simulink model "flightControlSystem2"  (R2019a)
settings: Solver=ode3  StartTime=0  StopTime=TFinal  FixedStep=Ts  RelTol=1e-3  EnableMultiTasking=on
InitFcn:
  | %生成模板
  | temp_Image = uint8(ones(120,160));
  | 
  | [m,n] = size(temp_Image);
  | angle = 10*pi/180;
  | 
  | left_point = 70;
  | right_point = 90;
  | j = 71;
  | for i = 1:50
  |     temp_left_point = floor(left_point - i*sin(angle));
  |     temp_right_point = floor(right_point + i*sin(angle));
  |     if temp_left_point < 1
  |         temp_left_point = 1;
  |     end
  |     if temp_right_point > 180
  |         temp_right_point = 180;
  |     end
  |     temp_Image(j,temp_left_point:temp_right_point) = 0;
  |     j = j+1;
  | end
undefined symbols (not defined in the file): codertarget, Controller, DiscIntNeverNeededParam, Discrete, Estimator, g, gray, init, pos_ref, Sensors, takeoff_flag, Time, Ts, Vehicle
libraries: simulink x60, visiontransforms x4, sharedtransform x3, ctrlSharedLib x2, visionsinks x2, sharedutil x1, visionanalysis x1, parrotlib x1
(part 3 of 3)

== matlab function flightControlSystem2/Control System/Path Planning/state_control ==
  data: line_sum_angle input; line_target input; line_flag input; drone_targetout output; circle_output input; drone_angle output; circle_flag input; drone_xyz input; yaw input; F1 data_store_memory; F2 data_store_memory; F3 data_store_memory
function [drone_targetout, drone_angle] = state_control(line_sum_angle, line_target, line_flag, circle_output, circle_flag, drone_xyz, yaw)

global F1 F2 F3

if line_flag == -1 && circle_flag ~= -1 && F1 ~= 2
    F1 = 1;
end

    
if F1 == 0
    % follow the line
    drone_target = line_target;
    drone_angle = line_sum_angle;
    target = [0,0,0]';
    sum_x = 0;
    sum_y = 0;
elseif F1 == 1
    % move toward the center of circle
    circle_output(1,1) = 160 - circle_output(1,1);
    circle_output(1,2) = 120 - circle_output(1,2);
    sum_y = circle_output(1,1)-80;
    sum_x = 60-circle_output(1,2);
     sum_x = sum_x;
     sum_y = -sum_y;
    temp = sqrt(sum_x^2 + sum_y^2);
    sum_x = sum_x/temp;
    sum_y = sum_y/temp;
    
    target = 0.15*9.4e-3*[sum_x;sum_y;0];
	distance = temp;
    
    drone_target = drone_xyz + target;
    drone_angle = double(yaw);
    
    if distance < 15
    F2  = F2 + 1;
    if F2 >= 1
       F1 = 2;
       F3 = drone_target;
    end
    
    end
    down = 0;
    drone_target(3) = drone_target(3) + down;
    
elseif F1 ==2
    % move down
    if circle_flag ~= -1
    circle_output(1,1) = 160 - circle_output(1,1);
    circle_output(1,2) = 120 - circle_output(1,2);
    sum_y = circle_output(1,1)-80;
    sum_x = 60-circle_output(1,2);
         sum_x = sum_x;
         sum_y = -sum_y;
        temp = sqrt(sum_x^2 + sum_y^2);
        sum_x = sum_x/temp;
        sum_y = sum_y/temp;

        target = 0.1*9.4e-3*[sum_x;sum_y;0];

%         if drone_xyz(3)>-0.5
%             target = [0,0,0]';
%         end
        
        drone_target = drone_xyz + target;
        drone_target = (drone_target + F3)/2;
        F3 = drone_target;
    else
        drone_target = F3;
    end
    
    sum_x = 0;
    sum_y = 0;
    
    drone_angle = double(yaw);
    drone_target = F3;

    down = 0.1;
    drone_target(3) = drone_target(3) + down;
    
% 	if drone_xyz(3)>-0.5
%         target = 0;
%     end
    
     F3 = drone_target;

else
    sum_x = 0;
    sum_y = 0;
    target = [0,0,0]';
    drone_target = F3;
    drone_angle = double(yaw);
end

drone_targetout = drone_target;
xxx = F2;
yyy = circle_flag;
ob1 = [sum_x,sum_y];

== matlab function flightControlSystem2/Control System/Path Planning/three_circles_control ==
  data: image_control_data input; drone_xyz input; line_sum_angle output; A1 data_store_memory; A3 data_store_memory; A2 data_store_memory; line_target output; yaw input; A4 data_store_memory; FLAG data_store_memory; index_model data_store_memory; B1 data_store_memory; B2 data_store_memory; B3 data_store_memory; B4 data_store_memory
function [line_sum_angle, line_target] = three_circles_control(image_control_data, drone_xyz, yaw)
Conv_coeff = image_control_data(1);
line_angle = image_control_data(2);

%% 定义
global A1 A2 A3 A4 FLAG index_model
global B1 B2 B3 B4

%% 角度
 line_angle = line_angle*0.7 + A1*0.1 + A2*0.1 + A3*0.1;
%%
% if abs(line_angle) > 1.5 
%     line_angle = 1.5;
% elseif abs(line_angle) <0.05
%     line_angle = 0;
% end

%% 分级调参
% 


% 一级档
if abs(line_angle) < 0.1
    angle_change = 0.15;
    speed_change = 7;
    
% 二级档
elseif abs(line_angle) < 0.2
   angle_change = 0.40;
   speed_change = 5.5;
   
% 三级档
elseif abs(line_angle) < 0.6
    angle_change = 0.5;
    speed_change = 3;
    
% 四级档
elseif abs(line_angle) < 1.2
    angle_change = 0.5;
    speed_change = 3;
    
% 五级档  
else 
    angle_change = 0.55;
    speed_change = 3;
    
end 

% speed_change = speed_change*0.8 + B1*0.1 + B2*0.1 ;

%% 1 + B3*0.1 + B4*0.1
% if abs(line_angle) < 0.1
%     angle_change = 0.15;
%     speed_change = 7;
%     
% % 二级档
% elseif abs(line_angle) < 0.4
%    angle_change = 0.40;
%    speed_change = 6;
   

%% 3

% % 一级档
% if abs(line_angle) < 0.1
%     angle_change = 0.15;
%     speed_change = 7;
%     
% % 二级档
% elseif abs(line_angle) < 0.2
%    angle_change = 0.40;
%    speed_change = 6;
%    
% % 三级档
% elseif abs(line_angle) < 0.6
%     angle_change = 0.5;
%     speed_change = 3;
%     
% % 四级档
% elseif abs(line_angle) < 1.2
%     angle_change = 0.5;
%     speed_change = 3;
%     
% % 五级档  
% else 
%     angle_change = 0.55;
%     speed_change = 3;
%     
% end 


% % 一级档
% if abs(line_angle) < 0.1
%     angle_change = 0.2;
%     speed_change = 7;
%     
% % 二级档
% elseif abs(line_angle) < 0.2
%    angle_change = 0.3;
%    speed_change = 7;
%    
% % 三级档
% elseif abs(line_angle) < 0.5
%     angle_change = 0.45;
%     speed_change = 3;
%     
% % 四级档
% elseif abs(line_angle) < 0.7
%     angle_change = 0.65;
%     speed_change = 4;
%     
% % 五级档  
% else 
%     angle_change = 0.55;
%     speed_change = 5;
%     
% end 

%%

% %% 分级调参
% % 
% 
% 
% % 一级档
% if abs(line_angle) < 0.1
%     angle_change = 0.15;
%     speed_change = 9;
%     
% % 二级档
% elseif abs(line_angle) < 0.2
%    angle_change = 0.25;
%    speed_change = 7;
%    
% % 三级档
% elseif abs(line_angle) < 0.6
%     angle_change = 0.35;
%     speed_change = 6;
%     
% % 四级档
% elseif abs(line_angle) < 0.7
%     angle_change = 0.45;
%     speed_change = 5;
%     
% % 五级档  
% else 
%     angle_change = 0.55;
%     speed_change = 5;
%     
% end 
%%
%% 函数调参
% angle_change = 0.667*abs(angle);
% speed_change = k*angle_change+ b;



%% 控制
if abs(drone_xyz(3)+1.1) > 0.1
    angle_change = 1;
end

sum_angle = double(yaw)+ angle_change *line_angle;

sum_x = cos(sum_angle);
sum_y = sin(sum_angle);
target = speed_change*Conv_coeff*[sum_x;sum_y;0];
target = drone_xyz + target;

% target(3) = -1.1;
if target(3) >= -1.1
    target(3) = target(3) - 0.1;
end

if abs(drone_xyz(3)+1.1) > 0.1
    target(1) = 0;
    target(2) = 0;
    
end
%     

%% 更新
A3 = A2;
A2 = A1;
A1 = line_angle;

B4 = B3;
B3 = B2;
B2 = B1;
B1 = speed_change;

line_sum_angle = sum_angle;
line_target = target;

== matlab function flightControlSystem2/Control System/Path Planning2/line_gravity_point ==
  data: Conv_coeff output; image_data input; A1 data_store_memory; A3 data_store_memory; A2 data_store_memory; center_gravity_area output; line_flag output
function [Conv_coeff,center_gravity_area,line_flag]  = center_gravity(image_data)
%% 找红色
r = image_data(1);
g = image_data(2);
b = image_data(3);
flag = 1;
Image = r;
index = g(:)>50 | b(:)>50;
Image(index) = 0;
Image = Image.*temp_Image;
[width,height] = size(Image);

%% 找路径
skeletonizedImage = bwmorph(Image, 'thin', inf);
edgeImage = bwperim(Image);
Image2 = bwperim(skeletonizedImage);

%% 求出转换系数
%等分处理,取众数，求出路宽,
%需要从图像的x,y方向上进行截取的原因是，为了保证无人机能转弯。
%因为后面求出了转换系数，只考虑x方向的话，到转弯处，转换系数会发现剧烈变化，从而影响输出。
% temp = zeros(26,1);
% k = 1;
% for i = 10:10:width-10 %水平方向取11个值
%     index = find(edgeImage(i,:) == 1);
%     if ~isempty(index)
%         temp(k) = max(index) - min(index);
%     else
%         temp(k) = k;
%     end
%      k = k+1;
% end
% for i = 10:10:height-10 %垂直方向取15个值
%     index = find(edgeImage(:,i) == 1);
%     if ~isempty(index)
%         temp(k) = max(index) - min(index);
%     else
%         temp(k) = k;
%     end
%      k = k+1;
% end
% road_image_length = mode(temp);
% 
% %转换系数，即真实距离与图像像素距离之比,一个像素对应的实际距离
% Conv_coeff = 0.15/road_image_length;
% if Conv_coeff > 0.01
%     Conv_coeff = 0.01;
% end
Conv_coeff = 9.4e-3;
%% 跟踪算法
Image_roi = Image2;
center_x = 60;
center_y = 80;

%%


cut = [45;50;55];

cut_XY = zeros(length(cut(:)),4);
for i = 1:length(cut_XY(:,1))
    cut_XY(i,1) = center_x - cut(i);
    cut_XY(i,2) = center_y - cut(i);
    cut_XY(i,3) = center_x + cut(i);
    cut_XY(i,4) = center_y + cut(i);
end

sum_vector = zeros(length(cut(:)),3);

for i = 1:length(cut_XY(:,1))
    I1 = Image_roi(cut_XY(i,1):cut_XY(i,3),cut_XY(i,2):cut_XY(i,4));
    index = find(I1(:)==1);
    position = zeros(length(index),3);
    I1_center_x = 1+cut(i);
    I1_center_y = 1+cut(i);
    if ~isempty(index)
        for k=1:length(index)
            [position(k,1),position(k,2)] = ind2sub(size(I1),index(k));
            position(k,1) = I1_center_x - position(k,1);
            position(k,2) = position(k,2) - I1_center_y;
            position(k,3) = sqrt((position(k,1))^2+(position(k,2))^2);
        end
        index1 = position(:,3) <= cut(i)+0.5 & position(:,3) >= cut(i)-0.5 & position(:,1) > 0;
        position = position(index1,:);
    end
    if ~isempty(index)
        if length(position(:,1))==1
            sum_vector(i,1) = position(1,1);
            sum_vector(i,2) = position(1,2);
            temp = sqrt(sum_vector(i,1)^2 + sum_vector(i,2)^2);
            sum_vector(i,1) = sum_vector(i,1)/temp;
            sum_vector(i,2) = sum_vector(i,2)/temp;
            sum_vector(i,3) = atan2(sum_vector(i,2),sum_vector(i,1));
        end
    end
end
% vector = 0.25*sum_vector(1,:)+0.5*sum_vector(2,:)+0.25*sum_vector(3,:);
vector = 0.3*sum_vector(1,:)+0.3*sum_vector(2,:)+0.4*sum_vector(3,:);
if abs(sum_vector(1,1)) < 1e-5 && abs(sum_vector(1,2)) < 1e-5
    flag = -1;
end
line = vector(3);
line_flag = flag;

== matlab function flightControlSystem2/Control System/Path Planning1/state_control ==
  data: center_gravity_point input; line_target input; line_flag input; drone_targetout output; circle_output input; drone_angle output; circle_flag input; drone_xyz input; yaw input; F1 data_store_memory; F2 data_store_memory; F3 data_store_memory
function [drone_targetout, drone_angle] = state_control(center_gravity_point, line_target, line_flag, circle_output, circle_flag, drone_xyz, yaw)

global F1 F2 F3

if line_flag == -1 && circle_flag ~= -1 && F1 ~= 2
    F1 = 1;
end

    
if F1 == 0
    % follow the line
    drone_target = line_target;
    drone_angle = line_sum_angle;
    target = [0,0,0]';
    sum_x = 0;
    sum_y = 0;
elseif F1 == 1
    % move toward the center of circle
    circle_output(1,1) = 160 - circle_output(1,1);
    circle_output(1,2) = 120 - circle_output(1,2);
    sum_y = circle_output(1,1)-80;
    sum_x = 60-circle_output(1,2);
     sum_x = sum_x;
     sum_y = -sum_y;
    temp = sqrt(sum_x^2 + sum_y^2);
    sum_x = sum_x/temp;
    sum_y = sum_y/temp;
    
    target = 0.15*9.4e-3*[sum_x;sum_y;0];
	distance = temp;
    
    drone_target = drone_xyz + target;
    drone_angle = double(yaw);
    
    if distance < 15
    F2  = F2 + 1;
    if F2 >= 1
       F1 = 2;
       F3 = drone_target;
    end
    
    end
    down = 0;
    drone_target(3) = drone_target(3) + down;
    
elseif F1 ==2
    % move down
    if circle_flag ~= -1
    circle_output(1,1) = 160 - circle_output(1,1);
    circle_output(1,2) = 120 - circle_output(1,2);
    sum_y = circle_output(1,1)-80;
    sum_x = 60-circle_output(1,2);
         sum_x = sum_x;
         sum_y = -sum_y;
        temp = sqrt(sum_x^2 + sum_y^2);
        sum_x = sum_x/temp;
        sum_y = sum_y/temp;

        target = 0.1*9.4e-3*[sum_x;sum_y;0];

%         if drone_xyz(3)>-0.5
%             target = [0,0,0]';
%         end
        
        drone_target = drone_xyz + target;
        drone_target = (drone_target + F3)/2;
        F3 = drone_target;
    else
        drone_target = F3;
    end
    
    sum_x = 0;
    sum_y = 0;
    
    drone_angle = double(yaw);
    drone_target = F3;

    down = 0.1;
    drone_target(3) = drone_target(3) + down;
    
% 	if drone_xyz(3)>-0.5
%         target = 0;
%     end
    
     F3 = drone_target;

else
    sum_x = 0;
    sum_y = 0;
    target = [0,0,0]';
    drone_target = F3;
    drone_angle = double(yaw);
end

drone_targetout = drone_target;
xxx = F2;
yyy = circle_flag;
ob1 = [sum_x,sum_y];

== matlab function flightControlSystem2/Control System/Path Planning1/center_gravity_control ==
  data: image_control_data input; drone_xyz input; center_gravity_point output; A1 data_store_memory; A3 data_store_memory; A2 data_store_memory; line_target output; yaw input; A4 data_store_memory; FLAG data_store_memory; index_model data_store_memory; B1 data_store_memory; B2 data_store_memory; B3 data_store_memory; B4 data_store_memory
function [center_gravity_point, line_target] = center_gravity_control(image_control_data, drone_xyz, yaw)
Conv_coeff = image_control_data(1);
line_angle = image_control_data(2);

%% 定义
global A1 A2 A3 A4 FLAG index_model
global B1 B2 B3 B4

%% 角度
 line_angle = line_angle*0.7 + A1*0.1 + A2*0.1 + A3*0.1;
%%
% if abs(line_angle) > 1.5 
%     line_angle = 1.5;
% elseif abs(line_angle) <0.05
%     line_angle = 0;
% end

%% 分级调参
% 


% 一级档
if abs(line_angle) < 0.1
    angle_change = 0.15;
    speed_change = 7;
    
% 二级档
elseif abs(line_angle) < 0.2
   angle_change = 0.40;
   speed_change = 5.5;
   
% 三级档
elseif abs(line_angle) < 0.6
    angle_change = 0.5;
    speed_change = 3;
    
% 四级档
elseif abs(line_angle) < 1.2
    angle_change = 0.5;
    speed_change = 3;
    
% 五级档  
else 
    angle_change = 0.55;
    speed_change = 3;
    
end 

% speed_change = speed_change*0.8 + B1*0.1 + B2*0.1 ;

%% 1 + B3*0.1 + B4*0.1
% if abs(line_angle) < 0.1
%     angle_change = 0.15;
%     speed_change = 7;
%     
% % 二级档
% elseif abs(line_angle) < 0.4
%    angle_change = 0.40;
%    speed_change = 6;
   

%% 3

% % 一级档
% if abs(line_angle) < 0.1
%     angle_change = 0.15;
%     speed_change = 7;
%     
% % 二级档
% elseif abs(line_angle) < 0.2
%    angle_change = 0.40;
%    speed_change = 6;
%    
% % 三级档
% elseif abs(line_angle) < 0.6
%     angle_change = 0.5;
%     speed_change = 3;
%     
% % 四级档
% elseif abs(line_angle) < 1.2
%     angle_change = 0.5;
%     speed_change = 3;
%     
% % 五级档  
% else 
%     angle_change = 0.55;
%     speed_change = 3;
%     
% end 


% % 一级档
% if abs(line_angle) < 0.1
%     angle_change = 0.2;
%     speed_change = 7;
%     
% % 二级档
% elseif abs(line_angle) < 0.2
%    angle_change = 0.3;
%    speed_change = 7;
%    
% % 三级档
% elseif abs(line_angle) < 0.5
%     angle_change = 0.45;
%     speed_change = 3;
%     
% % 四级档
% elseif abs(line_angle) < 0.7
%     angle_change = 0.65;
%     speed_change = 4;
%     
% % 五级档  
% else 
%     angle_change = 0.55;
%     speed_change = 5;
%     
% end 

%%

% %% 分级调参
% % 
% 
% 
% % 一级档
% if abs(line_angle) < 0.1
%     angle_change = 0.15;
%     speed_change = 9;
%     
% % 二级档
% elseif abs(line_angle) < 0.2
%    angle_change = 0.25;
%    speed_change = 7;
%    
% % 三级档
% elseif abs(line_angle) < 0.6
%     angle_change = 0.35;
%     speed_change = 6;
%     
% % 四级档
% elseif abs(line_angle) < 0.7
%     angle_change = 0.45;
%     speed_change = 5;
%     
% % 五级档  
% else 
%     angle_change = 0.55;
%     speed_change = 5;
%     
% end 
%%
%% 函数调参
% angle_change = 0.667*abs(angle);
% speed_change = k*angle_change+ b;



%% 控制
if abs(drone_xyz(3)+1.1) > 0.1
    angle_change = 1;
end

sum_angle = double(yaw)+ angle_change *line_angle;

sum_x = cos(sum_angle);
sum_y = sin(sum_angle);
target = speed_change*Conv_coeff*[sum_x;sum_y;0];
target = drone_xyz + target;

% target(3) = -1.1;
if target(3) >= -1.1
    target(3) = target(3) - 0.1;
end

if abs(drone_xyz(3)+1.1) > 0.1
    target(1) = 0;
    target(2) = 0;
    
end
%     

%% 更新
A3 = A2;
A2 = A1;
A1 = line_angle;

B4 = B3;
B3 = B2;
B2 = B1;
B1 = speed_change;

line_sum_angle = sum_angle;
line_target = target;

== matlab function flightControlSystem2/Control System/Path Planning2/state_control ==
  data: line_sum_angle input; line_flag input; drone_targetout output; circle_output input; drone_angle output; circle_flag input; drone_xyz input; yaw input; F1 data_store_memory; F2 data_store_memory; F3 data_store_memory
function [drone_targetout, drone_angle] = state_control(line_sum_angle, line_flag, circle_output, circle_flag, drone_xyz, yaw)

global F1 F2 F3

if line_flag == -1 && circle_flag ~= -1 && F1 ~= 2
    F1 = 1;
end

    
if F1 == 0
    % follow the line
    drone_target = line_target;
    drone_angle = line_sum_angle;
    target = [0,0,0]';
    sum_x = 0;
    sum_y = 0;
elseif F1 == 1
    % move toward the center of circle
    circle_output(1,1) = 160 - circle_output(1,1);
    circle_output(1,2) = 120 - circle_output(1,2);
    sum_y = circle_output(1,1)-80;
    sum_x = 60-circle_output(1,2);
     sum_x = sum_x;
     sum_y = -sum_y;
    temp = sqrt(sum_x^2 + sum_y^2);
    sum_x = sum_x/temp;
    sum_y = sum_y/temp;
    
    target = 0.15*9.4e-3*[sum_x;sum_y;0];
	distance = temp;
    
    drone_target = drone_xyz + target;
    drone_angle = double(yaw);
    
    if distance < 15
    F2  = F2 + 1;
    if F2 >= 1
       F1 = 2;
       F3 = drone_target;
    end
    
    end
    down = 0;
    drone_target(3) = drone_target(3) + down;
    
elseif F1 ==2
    % move down
    if circle_flag ~= -1
    circle_output(1,1) = 160 - circle_output(1,1);
    circle_output(1,2) = 120 - circle_output(1,2);
    sum_y = circle_output(1,1)-80;
    sum_x = 60-circle_output(1,2);
         sum_x = sum_x;
         sum_y = -sum_y;
        temp = sqrt(sum_x^2 + sum_y^2);
        sum_x = sum_x/temp;
        sum_y = sum_y/temp;

        target = 0.1*9.4e-3*[sum_x;sum_y;0];

%         if drone_xyz(3)>-0.5
%             target = [0,0,0]';
%         end
        
        drone_target = drone_xyz + target;
        drone_target = (drone_target + F3)/2;
        F3 = drone_target;
    else
        drone_target = F3;
    end
    
    sum_x = 0;
    sum_y = 0;
    
    drone_angle = double(yaw);
    drone_target = F3;

    down = 0.1;
    drone_target(3) = drone_target(3) + down;
    
% 	if drone_xyz(3)>-0.5
%         target = 0;
%     end
    
     F3 = drone_target;

else
    sum_x = 0;
    sum_y = 0;
    target = [0,0,0]';
    drone_target = F3;
    drone_angle = double(yaw);
end

drone_targetout = drone_target;
xxx = F2;
yyy = circle_flag;
ob1 = [sum_x,sum_y];

== matlab function flightControlSystem2/Control System/Path Planning2/random_points_control ==
  data: image_control_data input; drone_xyz input; random_point output; A1 data_store_memory; A3 data_store_memory; A2 data_store_memory; yaw input; A4 data_store_memory; FLAG data_store_memory; index_model data_store_memory; B1 data_store_memory; B2 data_store_memory; B3 data_store_memory; B4 data_store_memory
function random_point =  random_point_control(image_control_data, drone_xyz, yaw)
Conv_coeff = image_control_data(1);
line_angle = image_control_data(2);

%% 定义
global A1 A2 A3 A4 FLAG index_model
global B1 B2 B3 B4

%% 角度
 line_angle = line_angle*0.7 + A1*0.1 + A2*0.1 + A3*0.1;
%%
% if abs(line_angle) > 1.5 
%     line_angle = 1.5;
% elseif abs(line_angle) <0.05
%     line_angle = 0;
% end

%% 分级调参
% 


% 一级档
if abs(line_angle) < 0.1
    angle_change = 0.15;
    speed_change = 7;
    
% 二级档
elseif abs(line_angle) < 0.2
   angle_change = 0.40;
   speed_change = 5.5;
   
% 三级档
elseif abs(line_angle) < 0.6
    angle_change = 0.5;
    speed_change = 3;
    
% 四级档
elseif abs(line_angle) < 1.2
    angle_change = 0.5;
    speed_change = 3;
    
% 五级档  
else 
    angle_change = 0.55;
    speed_change = 3;
    
end 

% speed_change = speed_change*0.8 + B1*0.1 + B2*0.1 ;

%% 1 + B3*0.1 + B4*0.1
% if abs(line_angle) < 0.1
%     angle_change = 0.15;
%     speed_change = 7;
%     
% % 二级档
% elseif abs(line_angle) < 0.4
%    angle_change = 0.40;
%    speed_change = 6;
   

%% 3

% % 一级档
% if abs(line_angle) < 0.1
%     angle_change = 0.15;
%     speed_change = 7;
%     
% % 二级档
% elseif abs(line_angle) < 0.2
%    angle_change = 0.40;
%    speed_change = 6;
%    
% % 三级档
% elseif abs(line_angle) < 0.6
%     angle_change = 0.5;
%     speed_change = 3;
%     
% % 四级档
% elseif abs(line_angle) < 1.2
%     angle_change = 0.5;
%     speed_change = 3;
%     
% % 五级档  
% else 
%     angle_change = 0.55;
%     speed_change = 3;
%     
% end 


% % 一级档
% if abs(line_angle) < 0.1
%     angle_change = 0.2;
%     speed_change = 7;
%     
% % 二级档
% elseif abs(line_angle) < 0.2
%    angle_change = 0.3;
%    speed_change = 7;
%    
% % 三级档
% elseif abs(line_angle) < 0.5
%     angle_change = 0.45;
%     speed_change = 3;
%     
% % 四级档
% elseif abs(line_angle) < 0.7
%     angle_change = 0.65;
%     speed_change = 4;
%     
% % 五级档  
% else 
%     angle_change = 0.55;
%     speed_change = 5;
%     
% end 

%%

% %% 分级调参
% % 
% 
% 
% % 一级档
% if abs(line_angle) < 0.1
%     angle_change = 0.15;
%     speed_change = 9;
%     
% % 二级档
% elseif abs(line_angle) < 0.2
%    angle_change = 0.25;
%    speed_change = 7;
%    
% % 三级档
% elseif abs(line_angle) < 0.6
%     angle_change = 0.35;
%     speed_change = 6;
%     
% % 四级档
% elseif abs(line_angle) < 0.7
%     angle_change = 0.45;
%     speed_change = 5;
%     
% % 五级档  
% else 
%     angle_change = 0.55;
%     speed_change = 5;
%     
% end 
%%
%% 函数调参
% angle_change = 0.667*abs(angle);
% speed_change = k*angle_change+ b;



%% 控制
if abs(drone_xyz(3)+1.1) > 0.1
    angle_change = 1;
end

sum_angle = double(yaw)+ angle_change *line_angle;

sum_x = cos(sum_angle);
sum_y = sin(sum_angle);
target = speed_change*Conv_coeff*[sum_x;sum_y;0];
target = drone_xyz + target;

% target(3) = -1.1;
if target(3) >= -1.1
    target(3) = target(3) - 0.1;
end

if abs(drone_xyz(3)+1.1) > 0.1
    target(1) = 0;
    target(2) = 0;
    
end
%     

%% 更新
A3 = A2;
A2 = A1;
A1 = line_angle;

B4 = B3;
B3 = B2;
B2 = B1;
B1 = speed_change;

line_sum_angle = sum_angle;
line_target = target;

== matlab function flightControlSystem2/Image Processing System1/MATLAB Function1 ==
  data: R_stright output; origin output; R_Matrix input; y output; ab output
function [R_stright, origin,y,ab] = fcn(R_Matrix)
% a = simout.data(:,:,201);
% A = a>100;
% mc = mat2cell(A,repmat(10,1,12),repmat(10,1,16));
% MC = cellfun(@(x) sum(x(:)),mc);
R_numMatrix = zeros(12,16);
R_stright=R_Matrix(:,20:140);
for i=1:1:12
    for j=1:1:16
        m = 10*(i-1)+1;
        n = 10*(j-1)+1;
        for m = m:1:m+8
            for n = n:1:n+8
                if(R_Matrix(m,n) > 230)
                    R_numMatrix(i,j) = R_numMatrix(i,j)+1;
                end
            end
            n = 10*(j-1)+1;
        end
    end
end                                     %分区及像素计算完毕





%计算重心高斯矩阵
outOrigin=R_numMatrix;
Deno=sum(sum(R_numMatrix));
xFocus = (1:1:12) * R_numMatrix;
xFocus = sum(xFocus(:));
yFocus = R_numMatrix * (1:1:16)';
yFocus = sum(yFocus(:));
Focus = [xFocus yFocus]/Deno;

%四舍五入
if(mod(Focus(1),1)>0.5)
    Focus(1)=Focus(1)-mod(Focus(1),1)+1;
else
    Focus(1)=Focus(1)-mod(Focus(1),1);
end

if(mod(Focus(2),1)>0.5)
    Focus(2)=Focus(2)-mod(Focus(2),1)+1;
else
    Focus(2)=Focus(2)-mod(Focus(2),1);
end

a=ones(25,33);
weight_center = 4;
weight_minus = 0.1;
a(:,1:1:4)=ones(25,1)*((weight_center-15*weight_minus):weight_minus:(weight_center-12*weight_minus));
a(:,30:1:33)=ones(25,1)*((weight_center-12*weight_minus):-weight_minus:(weight_center-15*weight_minus));
for i=13:-1:1
   if(i==13) a(13,17)=weight_center;continue; end
   a((13-i):1:(13+i),(17-i))=weight_center-i*weight_minus;
   a((13-i):1:(13+i),(17+i))=weight_center-i*weight_minus;
   a((13-i),(17-i):1:(17+i))=weight_center-i*weight_minus;
   a((13+i),(17-i):1:(17+i))=weight_center-i*weight_minus;
end
a1=6;a2=7;
for i=1:1:16
    if(Focus(1)==i) a1=i;end
    if(Focus(2)==i) a2=i;end
end

weight=a((13-a1):1:(13+12-a1-1),(17-a2):1:(17+16-a2-1));
r=R_numMatrix .* weight;

origin=outOrigin;
y = r;
ab=[a1 a2];

== matlab function flightControlSystem2/Image Processing System1/line_detect ==
  data: Conv_coeff output; image_data input; line output; A1 data_store_memory; A3 data_store_memory; A2 data_store_memory; line_flag output
function [Conv_coeff, line, line_flag] = line_detect(image_data)
%% 找红色
r = image_data(1);
g = image_data(2);
b = image_data(3);
flag = 1;
Image = r;
index = g(:)>50 | b(:)>50;
Image(index) = 0;
Image = Image.*temp_Image;
[width,height] = size(Image);

%% 找路径
skeletonizedImage = bwmorph(Image, 'thin', inf);
edgeImage = bwperim(Image);
Image2 = bwperim(skeletonizedImage);

%% 求出转换系数
%等分处理,取众数，求出路宽,
%需要从图像的x,y方向上进行截取的原因是，为了保证无人机能转弯。
%因为后面求出了转换系数，只考虑x方向的话，到转弯处，转换系数会发现剧烈变化，从而影响输出。
% temp = zeros(26,1);
% k = 1;
% for i = 10:10:width-10 %水平方向取11个值
%     index = find(edgeImage(i,:) == 1);
%     if ~isempty(index)
%         temp(k) = max(index) - min(index);
%     else
%         temp(k) = k;
%     end
%      k = k+1;
% end
% for i = 10:10:height-10 %垂直方向取15个值
%     index = find(edgeImage(:,i) == 1);
%     if ~isempty(index)
%         temp(k) = max(index) - min(index);
%     else
%         temp(k) = k;
%     end
%      k = k+1;
% end
% road_image_length = mode(temp);
% 
% %转换系数，即真实距离与图像像素距离之比,一个像素对应的实际距离
% Conv_coeff = 0.15/road_image_length;
% if Conv_coeff > 0.01
%     Conv_coeff = 0.01;
% end
Conv_coeff = 9.4e-3;
%% 跟踪算法
Image_roi = Image2;
center_x = 60;
center_y = 80;

%%


cut = [45;50;55];

cut_XY = zeros(length(cut(:)),4);
for i = 1:length(cut_XY(:,1))
    cut_XY(i,1) = center_x - cut(i);
    cut_XY(i,2) = center_y - cut(i);
    cut_XY(i,3) = center_x + cut(i);
    cut_XY(i,4) = center_y + cut(i);
end

sum_vector = zeros(length(cut(:)),3);

for i = 1:length(cut_XY(:,1))
    I1 = Image_roi(cut_XY(i,1):cut_XY(i,3),cut_XY(i,2):cut_XY(i,4));
    index = find(I1(:)==1);
    position = zeros(length(index),3);
    I1_center_x = 1+cut(i);
    I1_center_y = 1+cut(i);
    if ~isempty(index)
        for k=1:length(index)
            [position(k,1),position(k,2)] = ind2sub(size(I1),index(k));
            position(k,1) = I1_center_x - position(k,1);
            position(k,2) = position(k,2) - I1_center_y;
            position(k,3) = sqrt((position(k,1))^2+(position(k,2))^2);
        end
        index1 = position(:,3) <= cut(i)+0.5 & position(:,3) >= cut(i)-0.5 & position(:,1) > 0;
        position = position(index1,:);
    end
    if ~isempty(index)
        if length(position(:,1))==1
            sum_vector(i,1) = position(1,1);
            sum_vector(i,2) = position(1,2);
            temp = sqrt(sum_vector(i,1)^2 + sum_vector(i,2)^2);
            sum_vector(i,1) = sum_vector(i,1)/temp;
            sum_vector(i,2) = sum_vector(i,2)/temp;
            sum_vector(i,3) = atan2(sum_vector(i,2),sum_vector(i,1));
        end
    end
end
% vector = 0.25*sum_vector(1,:)+0.5*sum_vector(2,:)+0.25*sum_vector(3,:);
vector = 0.3*sum_vector(1,:)+0.3*sum_vector(2,:)+0.4*sum_vector(3,:);
if abs(sum_vector(1,1)) < 1e-5 && abs(sum_vector(1,2)) < 1e-5
    flag = -1;
end
line = vector(3);
line_flag = flag;

== matlab function flightControlSystem2/Image Processing System/line_control ==
  data: Conv_coeff input; line_angle input; line_sum_angle output; A1 data_store_memory; A3 data_store_memory; A2 data_store_memory; line_target output; yaw input; drone_xyz input; A4 data_store_memory; FLAG data_store_memory; index_model data_store_memory; B1 data_store_memory; B2 data_store_memory; B3 data_store_memory; B4 data_store_memory
function [line_sum_angle, line_target] = line_control(Conv_coeff, line_angle, yaw, drone_xyz)
%% 定义
global A1 A2 A3 A4 FLAG index_model
global B1 B2 B3 B4

%% 角度
 line_angle = line_angle*0.7 + A1*0.1 + A2*0.1 + A3*0.1;
%%
% if abs(line_angle) > 1.5 
%     line_angle = 1.5;
% elseif abs(line_angle) <0.05
%     line_angle = 0;
% end

%% 分级调参
% 


% 一级档
if abs(line_angle) < 0.1
    angle_change = 0.15;
    speed_change = 7;
    
% 二级档
elseif abs(line_angle) < 0.2
   angle_change = 0.40;
   speed_change = 5.5;
   
% 三级档
elseif abs(line_angle) < 0.6
    angle_change = 0.5;
    speed_change = 3;
    
% 四级档
elseif abs(line_angle) < 1.2
    angle_change = 0.5;
    speed_change = 3;
    
% 五级档  
else 
    angle_change = 0.55;
    speed_change = 3;
    
end 

% speed_change = speed_change*0.8 + B1*0.1 + B2*0.1 ;

%% 1 + B3*0.1 + B4*0.1
% if abs(line_angle) < 0.1
%     angle_change = 0.15;
%     speed_change = 7;
%     
% % 二级档
% elseif abs(line_angle) < 0.4
%    angle_change = 0.40;
%    speed_change = 6;
   

%% 3

% % 一级档
% if abs(line_angle) < 0.1
%     angle_change = 0.15;
%     speed_change = 7;
%     
% % 二级档
% elseif abs(line_angle) < 0.2
%    angle_change = 0.40;
%    speed_change = 6;
%    
% % 三级档
% elseif abs(line_angle) < 0.6
%     angle_change = 0.5;
%     speed_change = 3;
%     
% % 四级档
% elseif abs(line_angle) < 1.2
%     angle_change = 0.5;
%     speed_change = 3;
%     
% % 五级档  
% else 
%     angle_change = 0.55;
%     speed_change = 3;
%     
% end 


% % 一级档
% if abs(line_angle) < 0.1
%     angle_change = 0.2;
%     speed_change = 7;
%     
% % 二级档
% elseif abs(line_angle) < 0.2
%    angle_change = 0.3;
%    speed_change = 7;
%    
% % 三级档
% elseif abs(line_angle) < 0.5
%     angle_change = 0.45;
%     speed_change = 3;
%     
% % 四级档
% elseif abs(line_angle) < 0.7
%     angle_change = 0.65;
%     speed_change = 4;
%     
% % 五级档  
% else 
%     angle_change = 0.55;
%     speed_change = 5;
%     
% end 

%%

% %% 分级调参
% % 
% 
% 
% % 一级档
% if abs(line_angle) < 0.1
%     angle_change = 0.15;
%     speed_change = 9;
%     
% % 二级档
% elseif abs(line_angle) < 0.2
%    angle_change = 0.25;
%    speed_change = 7;
%    
% % 三级档
% elseif abs(line_angle) < 0.6
%     angle_change = 0.35;
%     speed_change = 6;
%     
% % 四级档
% elseif abs(line_angle) < 0.7
%     angle_change = 0.45;
%     speed_change = 5;
%     
% % 五级档  
% else 
%     angle_change = 0.55;
%     speed_change = 5;
%     
% end 
%%
%% 函数调参
% angle_change = 0.667*abs(angle);
% speed_change = k*angle_change+ b;



%% 控制
if abs(drone_xyz(3)+1.1) > 0.1
    angle_change = 1;
end

sum_angle = double(yaw)+ angle_change *line_angle;

sum_x = cos(sum_angle);
sum_y = sin(sum_angle);
target = speed_change*Conv_coeff*[sum_x;sum_y;0];
target = drone_xyz + target;

% target(3) = -1.1;
if target(3) >= -1.1
    target(3) = target(3) - 0.1;
end

if abs(drone_xyz(3)+1.1) > 0.1
    target(1) = 0;
    target(2) = 0;
    
end
%     

%% 更新
A3 = A2;
A2 = A1;
A1 = line_angle;

B4 = B3;
B3 = B2;
B2 = B1;
B1 = speed_change;

line_sum_angle = sum_angle;
line_target = target;

== matlab function flightControlSystem2/Image Processing System/state_control ==
  data: line_sum_angle input; line_target input; line_flag input; drone_targetout output; circle_output input; drone_angle output; circle_flag input; drone_xyz input; yaw input; F1 data_store_memory; F2 data_store_memory; F3 data_store_memory
function [drone_targetout, drone_angle] = state_control(line_sum_angle, line_target, line_flag, circle_output, circle_flag, drone_xyz, yaw)

global F1 F2 F3

if line_flag == -1 && circle_flag ~= -1 && F1 ~= 2
    F1 = 1;
end

    
if F1 == 0
    % follow the line
    drone_target = line_target;
    drone_angle = line_sum_angle;
    target = [0,0,0]';
    sum_x = 0;
    sum_y = 0;
elseif F1 == 1
    % move toward the center of circle
    circle_output(1,1) = 160 - circle_output(1,1);
    circle_output(1,2) = 120 - circle_output(1,2);
    sum_y = circle_output(1,1)-80;
    sum_x = 60-circle_output(1,2);
     sum_x = sum_x;
     sum_y = -sum_y;
    temp = sqrt(sum_x^2 + sum_y^2);
    sum_x = sum_x/temp;
    sum_y = sum_y/temp;
    
    target = 0.15*9.4e-3*[sum_x;sum_y;0];
	distance = temp;
    
    drone_target = drone_xyz + target;
    drone_angle = double(yaw);
    
    if distance < 15
    F2  = F2 + 1;
    if F2 >= 1
       F1 = 2;
       F3 = drone_target;
    end
    
    end
    down = 0;
    drone_target(3) = drone_target(3) + down;
    
elseif F1 ==2
    % move down
    if circle_flag ~= -1
    circle_output(1,1) = 160 - circle_output(1,1);
    circle_output(1,2) = 120 - circle_output(1,2);
    sum_y = circle_output(1,1)-80;
    sum_x = 60-circle_output(1,2);
         sum_x = sum_x;
         sum_y = -sum_y;
        temp = sqrt(sum_x^2 + sum_y^2);
        sum_x = sum_x/temp;
        sum_y = sum_y/temp;

        target = 0.1*9.4e-3*[sum_x;sum_y;0];

%         if drone_xyz(3)>-0.5
%             target = [0,0,0]';
%         end
        
        drone_target = drone_xyz + target;
        drone_target = (drone_target + F3)/2;
        F3 = drone_target;
    else
        drone_target = F3;
    end
    
    sum_x = 0;
    sum_y = 0;
    
    drone_angle = double(yaw);
    drone_target = F3;

    down = 0.1;
    drone_target(3) = drone_target(3) + down;
    
% 	if drone_xyz(3)>-0.5
%         target = 0;
%     end
    
     F3 = drone_target;

else
    sum_x = 0;
    sum_y = 0;
    target = [0,0,0]';
    drone_target = F3;
    drone_angle = double(yaw);
end

drone_targetout = drone_target;
xxx = F2;
yyy = circle_flag;
ob1 = [sum_x,sum_y];

== matlab function flightControlSystem2/Image Processing System/line_gravity_point ==
  data: Conv_coeff output; image_data input; A1 data_store_memory; A3 data_store_memory; A2 data_store_memory; center_gravity_area output; line_flag output
function [Conv_coeff,center_gravity_area,line_flag]  = center_gravity(image_data)
%% 找红色
r = image_data(1);
g = image_data(2);
b = image_data(3);
flag = 1;
Image = r;
index = g(:)>50 | b(:)>50;
Image(index) = 0;
Image = Image.*temp_Image;
[width,height] = size(Image);

%% 找路径
skeletonizedImage = bwmorph(Image, 'thin', inf);
edgeImage = bwperim(Image);
Image2 = bwperim(skeletonizedImage);

%% 求出转换系数
%等分处理,取众数，求出路宽,
%需要从图像的x,y方向上进行截取的原因是，为了保证无人机能转弯。
%因为后面求出了转换系数，只考虑x方向的话，到转弯处，转换系数会发现剧烈变化，从而影响输出。
% temp = zeros(26,1);
% k = 1;
% for i = 10:10:width-10 %水平方向取11个值
%     index = find(edgeImage(i,:) == 1);
%     if ~isempty(index)
%         temp(k) = max(index) - min(index);
%     else
%         temp(k) = k;
%     end
%      k = k+1;
% end
% for i = 10:10:height-10 %垂直方向取15个值
%     index = find(edgeImage(:,i) == 1);
%     if ~isempty(index)
%         temp(k) = max(index) - min(index);
%     else
%         temp(k) = k;
%     end
%      k = k+1;
% end
% road_image_length = mode(temp);
% 
% %转换系数，即真实距离与图像像素距离之比,一个像素对应的实际距离
% Conv_coeff = 0.15/road_image_length;
% if Conv_coeff > 0.01
%     Conv_coeff = 0.01;
% end
Conv_coeff = 9.4e-3;
%% 跟踪算法
Image_roi = Image2;
center_x = 60;
center_y = 80;

%%


cut = [45;50;55];

cut_XY = zeros(length(cut(:)),4);
for i = 1:length(cut_XY(:,1))
    cut_XY(i,1) = center_x - cut(i);
    cut_XY(i,2) = center_y - cut(i);
    cut_XY(i,3) = center_x + cut(i);
    cut_XY(i,4) = center_y + cut(i);
end

sum_vector = zeros(length(cut(:)),3);

for i = 1:length(cut_XY(:,1))
    I1 = Image_roi(cut_XY(i,1):cut_XY(i,3),cut_XY(i,2):cut_XY(i,4));
    index = find(I1(:)==1);
    position = zeros(length(index),3);
    I1_center_x = 1+cut(i);
    I1_center_y = 1+cut(i);
    if ~isempty(index)
        for k=1:length(index)
            [position(k,1),position(k,2)] = ind2sub(size(I1),index(k));
            position(k,1) = I1_center_x - position(k,1);
            position(k,2) = position(k,2) - I1_center_y;
            position(k,3) = sqrt((position(k,1))^2+(position(k,2))^2);
        end
        index1 = position(:,3) <= cut(i)+0.5 & position(:,3) >= cut(i)-0.5 & position(:,1) > 0;
        position = position(index1,:);
    end
    if ~isempty(index)
        if length(position(:,1))==1
            sum_vector(i,1) = position(1,1);
            sum_vector(i,2) = position(1,2);
            temp = sqrt(sum_vector(i,1)^2 + sum_vector(i,2)^2);
            sum_vector(i,1) = sum_vector(i,1)/temp;
            sum_vector(i,2) = sum_vector(i,2)/temp;
            sum_vector(i,3) = atan2(sum_vector(i,2),sum_vector(i,1));
        end
    end
end
% vector = 0.25*sum_vector(1,:)+0.5*sum_vector(2,:)+0.25*sum_vector(3,:);
vector = 0.3*sum_vector(1,:)+0.3*sum_vector(2,:)+0.4*sum_vector(3,:);
if abs(sum_vector(1,1)) < 1e-5 && abs(sum_vector(1,2)) < 1e-5
    flag = -1;
end
line = vector(3);
line_flag = flag;

== matlab function flightControlSystem2/Image Processing System2/line_control ==
  data: Conv_coeff input; line_angle input; line_sum_angle output; A1 data_store_memory; A3 data_store_memory; A2 data_store_memory; line_target output; yaw input; drone_xyz input; A4 data_store_memory; FLAG data_store_memory; index_model data_store_memory; B1 data_store_memory; B2 data_store_memory; B3 data_store_memory; B4 data_store_memory
function [line_sum_angle, line_target] = line_control(Conv_coeff, line_angle, yaw, drone_xyz)
%% 定义
global A1 A2 A3 A4 FLAG index_model
global B1 B2 B3 B4

%% 角度
 line_angle = line_angle*0.7 + A1*0.1 + A2*0.1 + A3*0.1;
%%
% if abs(line_angle) > 1.5 
%     line_angle = 1.5;
% elseif abs(line_angle) <0.05
%     line_angle = 0;
% end

%% 分级调参
% 


% 一级档
if abs(line_angle) < 0.1
    angle_change = 0.15;
    speed_change = 7;
    
% 二级档
elseif abs(line_angle) < 0.2
   angle_change = 0.40;
   speed_change = 5.5;
   
% 三级档
elseif abs(line_angle) < 0.6
    angle_change = 0.5;
    speed_change = 3;
    
% 四级档
elseif abs(line_angle) < 1.2
    angle_change = 0.5;
    speed_change = 3;
    
% 五级档  
else 
    angle_change = 0.55;
    speed_change = 3;
    
end 

% speed_change = speed_change*0.8 + B1*0.1 + B2*0.1 ;

%% 1 + B3*0.1 + B4*0.1
% if abs(line_angle) < 0.1
%     angle_change = 0.15;
%     speed_change = 7;
%     
% % 二级档
% elseif abs(line_angle) < 0.4
%    angle_change = 0.40;
%    speed_change = 6;
   

%% 3

% % 一级档
% if abs(line_angle) < 0.1
%     angle_change = 0.15;
%     speed_change = 7;
%     
% % 二级档
% elseif abs(line_angle) < 0.2
%    angle_change = 0.40;
%    speed_change = 6;
%    
% % 三级档
% elseif abs(line_angle) < 0.6
%     angle_change = 0.5;
%     speed_change = 3;
%     
% % 四级档
% elseif abs(line_angle) < 1.2
%     angle_change = 0.5;
%     speed_change = 3;
%     
% % 五级档  
% else 
%     angle_change = 0.55;
%     speed_change = 3;
%     
% end 


% % 一级档
% if abs(line_angle) < 0.1
%     angle_change = 0.2;
%     speed_change = 7;
%     
% % 二级档
% elseif abs(line_angle) < 0.2
%    angle_change = 0.3;
%    speed_change = 7;
%    
% % 三级档
% elseif abs(line_angle) < 0.5
%     angle_change = 0.45;
%     speed_change = 3;
%     
% % 四级档
% elseif abs(line_angle) < 0.7
%     angle_change = 0.65;
%     speed_change = 4;
%     
% % 五级档  
% else 
%     angle_change = 0.55;
%     speed_change = 5;
%     
% end 

%%

% %% 分级调参
% % 
% 
% 
% % 一级档
% if abs(line_angle) < 0.1
%     angle_change = 0.15;
%     speed_change = 9;
%     
% % 二级档
% elseif abs(line_angle) < 0.2
%    angle_change = 0.25;
%    speed_change = 7;
%    
% % 三级档
% elseif abs(line_angle) < 0.6
%     angle_change = 0.35;
%     speed_change = 6;
%     
% % 四级档
% elseif abs(line_angle) < 0.7
%     angle_change = 0.45;
%     speed_change = 5;
%     
% % 五级档  
% else 
%     angle_change = 0.55;
%     speed_change = 5;
%     
% end 
%%
%% 函数调参
% angle_change = 0.667*abs(angle);
% speed_change = k*angle_change+ b;



%% 控制
if abs(drone_xyz(3)+1.1) > 0.1
    angle_change = 1;
end

sum_angle = double(yaw)+ angle_change *line_angle;

sum_x = cos(sum_angle);
sum_y = sin(sum_angle);
target = speed_change*Conv_coeff*[sum_x;sum_y;0];
target = drone_xyz + target;

% target(3) = -1.1;
if target(3) >= -1.1
    target(3) = target(3) - 0.1;
end

if abs(drone_xyz(3)+1.1) > 0.1
    target(1) = 0;
    target(2) = 0;
    
end
%     

%% 更新
A3 = A2;
A2 = A1;
A1 = line_angle;

B4 = B3;
B3 = B2;
B2 = B1;
B1 = speed_change;

line_sum_angle = sum_angle;
line_target = target;

== matlab function flightControlSystem2/Image Processing System2/line_detect ==
  data: Conv_coeff output; image_data input; line output; A1 data_store_memory; A3 data_store_memory; A2 data_store_memory; line_flag output; temp_Image input
function [Conv_coeff, line, line_flag] = line_detect(image_data,temp_Image)
%% 找红色
r = image_data(1);
g = image_data(2);
b = image_data(3);
flag = 1;
Image = r;
index = g(:)>50 | b(:)>50;
Image(index) = 0;
Image = Image.*temp_Image;
[width,height] = size(Image);

%% 找路径
skeletonizedImage = bwmorph(Image, 'thin', inf);
edgeImage = bwperim(Image);
Image2 = bwperim(skeletonizedImage);

%% 求出转换系数
%等分处理,取众数，求出路宽,
%需要从图像的x,y方向上进行截取的原因是，为了保证无人机能转弯。
%因为后面求出了转换系数，只考虑x方向的话，到转弯处，转换系数会发现剧烈变化，从而影响输出。
% temp = zeros(26,1);
% k = 1;
% for i = 10:10:width-10 %水平方向取11个值
%     index = find(edgeImage(i,:) == 1);
%     if ~isempty(index)
%         temp(k) = max(index) - min(index);
%     else
%         temp(k) = k;
%     end
%      k = k+1;
% end
% for i = 10:10:height-10 %垂直方向取15个值
%     index = find(edgeImage(:,i) == 1);
%     if ~isempty(index)
%         temp(k) = max(index) - min(index);
%     else
%         temp(k) = k;
%     end
%      k = k+1;
% end
% road_image_length = mode(temp);
% 
% %转换系数，即真实距离与图像像素距离之比,一个像素对应的实际距离
% Conv_coeff = 0.15/road_image_length;
% if Conv_coeff > 0.01
%     Conv_coeff = 0.01;
% end
Conv_coeff = 9.4e-3;
%% 跟踪算法
Image_roi = Image2;
center_x = 60;
center_y = 80;

%%


cut = [45;50;55];

cut_XY = zeros(length(cut(:)),4);
for i = 1:length(cut_XY(:,1))
    cut_XY(i,1) = center_x - cut(i);
    cut_XY(i,2) = center_y - cut(i);
    cut_XY(i,3) = center_x + cut(i);
    cut_XY(i,4) = center_y + cut(i);
end

sum_vector = zeros(length(cut(:)),3);

for i = 1:length(cut_XY(:,1))
    I1 = Image_roi(cut_XY(i,1):cut_XY(i,3),cut_XY(i,2):cut_XY(i,4));
    index = find(I1(:)==1);
    position = zeros(length(index),3);
    I1_center_x = 1+cut(i);
    I1_center_y = 1+cut(i);
    if ~isempty(index)
        for k=1:length(index)
            [position(k,1),position(k,2)] = ind2sub(size(I1),index(k));
            position(k,1) = I1_center_x - position(k,1);
            position(k,2) = position(k,2) - I1_center_y;
            position(k,3) = sqrt((position(k,1))^2+(position(k,2))^2);
        end
        index1 = position(:,3) <= cut(i)+0.5 & position(:,3) >= cut(i)-0.5 & position(:,1) > 0;
        position = position(index1,:);
    end
    if ~isempty(index)
        if length(position(:,1))==1
            sum_vector(i,1) = position(1,1);
            sum_vector(i,2) = position(1,2);
            temp = sqrt(sum_vector(i,1)^2 + sum_vector(i,2)^2);
            sum_vector(i,1) = sum_vector(i,1)/temp;
            sum_vector(i,2) = sum_vector(i,2)/temp;
            sum_vector(i,3) = atan2(sum_vector(i,2),sum_vector(i,1));
        end
    end
end
% vector = 0.25*sum_vector(1,:)+0.5*sum_vector(2,:)+0.25*sum_vector(3,:);
vector = 0.3*sum_vector(1,:)+0.3*sum_vector(2,:)+0.4*sum_vector(3,:);
if abs(sum_vector(1,1)) < 1e-5 && abs(sum_vector(1,2)) < 1e-5
    flag = -1;
end
line = vector(3);
line_flag = flag;

== matlab function flightControlSystem2/Image Processing System2/line_gravity_point ==
  data: Conv_coeff output; image_data input; A1 data_store_memory; A3 data_store_memory; A2 data_store_memory; center_gravity_area output; line_flag output
function [Conv_coeff,center_gravity_area,line_flag]  = center_gravity(image_data)
%% 找红色
r = image_data(1);
g = image_data(2);
b = image_data(3);
flag = 1;
Image = r;
index = g(:)>50 | b(:)>50;
Image(index) = 0;
Image = Image.*temp_Image;
[width,height] = size(Image);

%% 找路径
skeletonizedImage = bwmorph(Image, 'thin', inf);
edgeImage = bwperim(Image);
Image2 = bwperim(skeletonizedImage);

%% 求出转换系数
%等分处理,取众数，求出路宽,
%需要从图像的x,y方向上进行截取的原因是，为了保证无人机能转弯。
%因为后面求出了转换系数，只考虑x方向的话，到转弯处，转换系数会发现剧烈变化，从而影响输出。
% temp = zeros(26,1);
% k = 1;
% for i = 10:10:width-10 %水平方向取11个值
%     index = find(edgeImage(i,:) == 1);
%     if ~isempty(index)
%         temp(k) = max(index) - min(index);
%     else
%         temp(k) = k;
%     end
%      k = k+1;
% end
% for i = 10:10:height-10 %垂直方向取15个值
%     index = find(edgeImage(:,i) == 1);
%     if ~isempty(index)
%         temp(k) = max(index) - min(index);
%     else
%         temp(k) = k;
%     end
%      k = k+1;
% end
% road_image_length = mode(temp);
% 
% %转换系数，即真实距离与图像像素距离之比,一个像素对应的实际距离
% Conv_coeff = 0.15/road_image_length;
% if Conv_coeff > 0.01
%     Conv_coeff = 0.01;
% end
Conv_coeff = 9.4e-3;
%% 跟踪算法
Image_roi = Image2;
center_x = 60;
center_y = 80;

%%


cut = [45;50;55];

cut_XY = zeros(length(cut(:)),4);
for i = 1:length(cut_XY(:,1))
    cut_XY(i,1) = center_x - cut(i);
    cut_XY(i,2) = center_y - cut(i);
    cut_XY(i,3) = center_x + cut(i);
    cut_XY(i,4) = center_y + cut(i);
end

sum_vector = zeros(length(cut(:)),3);

for i = 1:length(cut_XY(:,1))
    I1 = Image_roi(cut_XY(i,1):cut_XY(i,3),cut_XY(i,2):cut_XY(i,4));
    index = find(I1(:)==1);
    position = zeros(length(index),3);
    I1_center_x = 1+cut(i);
    I1_center_y = 1+cut(i);
    if ~isempty(index)
        for k=1:length(index)
            [position(k,1),position(k,2)] = ind2sub(size(I1),index(k));
            position(k,1) = I1_center_x - position(k,1);
            position(k,2) = position(k,2) - I1_center_y;
            position(k,3) = sqrt((position(k,1))^2+(position(k,2))^2);
        end
        index1 = position(:,3) <= cut(i)+0.5 & position(:,3) >= cut(i)-0.5 & position(:,1) > 0;
        position = position(index1,:);
    end
    if ~isempty(index)
        if length(position(:,1))==1
            sum_vector(i,1) = position(1,1);
            sum_vector(i,2) = position(1,2);
            temp = sqrt(sum_vector(i,1)^2 + sum_vector(i,2)^2);
            sum_vector(i,1) = sum_vector(i,1)/temp;
            sum_vector(i,2) = sum_vector(i,2)/temp;
            sum_vector(i,3) = atan2(sum_vector(i,2),sum_vector(i,1));
        end
    end
end
% vector = 0.25*sum_vector(1,:)+0.5*sum_vector(2,:)+0.25*sum_vector(3,:);
vector = 0.3*sum_vector(1,:)+0.3*sum_vector(2,:)+0.4*sum_vector(3,:);
if abs(sum_vector(1,1)) < 1e-5 && abs(sum_vector(1,2)) < 1e-5
    flag = -1;
end
line = vector(3);
line_flag = flag;

== matlab function flightControlSystem2/Image Processing System2/state_control ==
  data: line_sum_angle input; line_target input; line_flag input; drone_targetout output; circle_output input; drone_angle output; circle_flag input; drone_xyz input; yaw input; F1 data_store_memory; F2 data_store_memory; F3 data_store_memory
function [drone_targetout, drone_angle] = state_control(line_sum_angle, line_target, line_flag, circle_output, circle_flag, drone_xyz, yaw)

global F1 F2 F3

if line_flag == -1 && circle_flag ~= -1 && F1 ~= 2
    F1 = 1;
end

    
if F1 == 0
    % follow the line
    drone_target = line_target;
    drone_angle = line_sum_angle;
    target = [0,0,0]';
    sum_x = 0;
    sum_y = 0;
elseif F1 == 1
    % move toward the center of circle
    circle_output(1,1) = 160 - circle_output(1,1);
    circle_output(1,2) = 120 - circle_output(1,2);
    sum_y = circle_output(1,1)-80;
    sum_x = 60-circle_output(1,2);
     sum_x = sum_x;
     sum_y = -sum_y;
    temp = sqrt(sum_x^2 + sum_y^2);
    sum_x = sum_x/temp;
    sum_y = sum_y/temp;
    
    target = 0.15*9.4e-3*[sum_x;sum_y;0];
	distance = temp;
    
    drone_target = drone_xyz + target;
    drone_angle = double(yaw);
    
    if distance < 15
    F2  = F2 + 1;
    if F2 >= 1
       F1 = 2;
       F3 = drone_target;
    end
    
    end
    down = 0;
    drone_target(3) = drone_target(3) + down;
    
elseif F1 ==2
    % move down
    if circle_flag ~= -1
    circle_output(1,1) = 160 - circle_output(1,1);
    circle_output(1,2) = 120 - circle_output(1,2);
    sum_y = circle_output(1,1)-80;
    sum_x = 60-circle_output(1,2);
         sum_x = sum_x;
         sum_y = -sum_y;
        temp = sqrt(sum_x^2 + sum_y^2);
        sum_x = sum_x/temp;
        sum_y = sum_y/temp;

        target = 0.1*9.4e-3*[sum_x;sum_y;0];

%         if drone_xyz(3)>-0.5
%             target = [0,0,0]';
%         end
        
        drone_target = drone_xyz + target;
        drone_target = (drone_target + F3)/2;
        F3 = drone_target;
    else
        drone_target = F3;
    end
    
    sum_x = 0;
    sum_y = 0;
    
    drone_angle = double(yaw);
    drone_target = F3;

    down = 0.1;
    drone_target(3) = drone_target(3) + down;
    
% 	if drone_xyz(3)>-0.5
%         target = 0;
%     end
    
     F3 = drone_target;

else
    sum_x = 0;
    sum_y = 0;
    target = [0,0,0]';
    drone_target = F3;
    drone_angle = double(yaw);
end

drone_targetout = drone_target;
xxx = F2;
yyy = circle_flag;
ob1 = [sum_x,sum_y];
